simulink model "CBF_for_KinematicControl_UR3"  (R2024a)
settings: Solver=FixedStepAuto  StartTime=0.0  StopTime=Tf  FixedStep=Ts  RelTol=1e-3
undefined symbols (not defined in the file): config, d, InitAng, InitPos, lambda, Ts, x_obs
libraries: robotmaniplib x3, matrix_library x2, slctrl_constraint x1
settings Model: Creator=bumyong  LastModifiedBy=bumyong

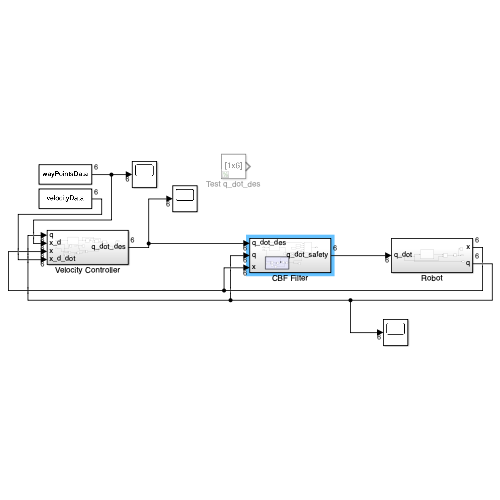
[thumbnail: Simulink's stored preview of the top-level diagram]
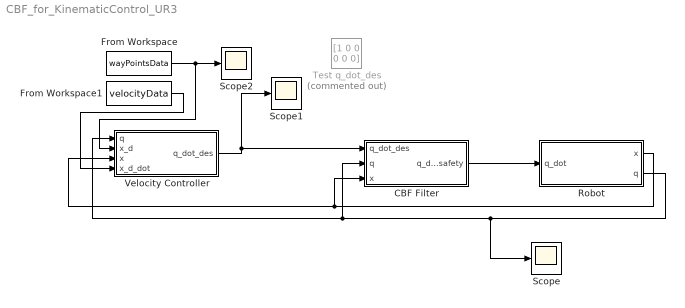
== system CBF_for_KinematicControl_UR3 ==
  CBF Filter : Subsystem
  From Workspace : FromWorkspace  VariableName=wayPointsData  Interpolate=off  OutputAfterFinalValue=Holding final value
  From Workspace1 : FromWorkspace  VariableName=velocityData  Interpolate=off  OutputAfterFinalValue=Holding final value
  Robot : Subsystem
  Scope : Scope
  Scope1 : Scope
  Scope2 : Scope
  Test q_dot_des : Constant  Commented=on  Value=[1 0 0 0 0 0]
  Velocity Controller : Subsystem
  wires:
  Robot/2(q) -> Scope/1, Velocity Controller/1(q), CBF Filter/2(q)
  Velocity Controller/1(q_dot_des) -> CBF Filter/1(q_dot_des), Scope1/1
  Robot/1(x) -> CBF Filter/3(x), Velocity Controller/3(x)
  From Workspace/1 -> Velocity Controller/2(x_d), Scope2/1
  From Workspace1/1 -> Velocity Controller/4(x_d_dot)
  CBF Filter/1(q_dot_safety) -> Robot/1(q_dot)

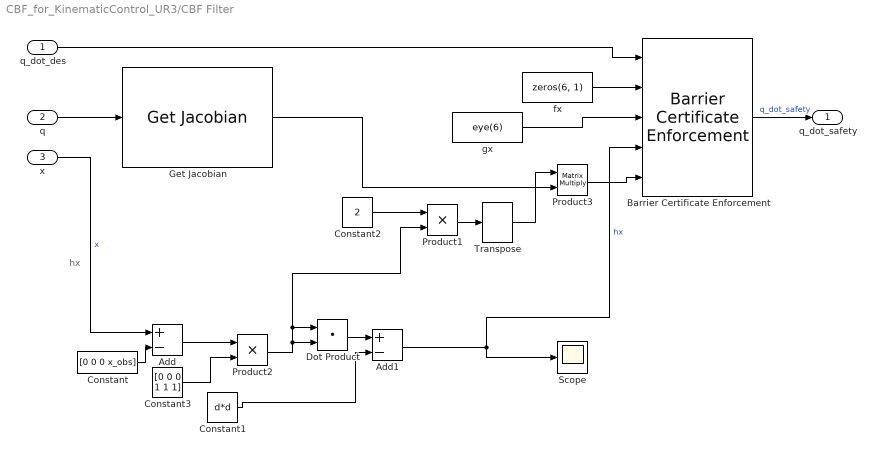
== system CBF_for_KinematicControl_UR3/CBF Filter ==
  note: hx
  q_dot_des : Inport
  q : Inport  Port=2
  x : Inport  Port=3
  Add : Sum  Inputs=+-
  Add1 : Sum  Inputs=+-
  Barrier Certificate Enforcement : slctrl_constraint/Barrier Certificate Enforcement  nx=6  nu=6  nc=1  gamma=gamma  beta=1  external_umax=off  external_umin=off  Ts=Ts  maxiter=200  tol=1e-6  output_exitflag=off
      settings: LibrarySourceBlock=slctrlblks/Constraint Control/Barrier Certificate Enforcement
  Constant : Constant  Value=[0 0 0 x_obs]
  Constant1 : Constant  Value=d*d
  Constant2 : Constant  Value=2
  Constant3 : Constant  Value=[0 0 0 1 1 1]
  Dot Product : DotProduct  OutDataTypeStr=Inherit: Inherit via internal rule
  Get Jacobian : robotmaniplib/Get Jacobian  RigidBodyTree=robot  EndEffector=tool0  SimulateUsing=Interpreted execution
  Product1 : Product
  Product2 : Product
  Product3 : Product  Multiplication=Matrix(*)
  Scope : Scope
  Transpose : matrix_library/Transpose
  fx : Constant  Value=zeros(6, 1)
  gx : Constant  Value=eye(6)
  q_dot_safety : Outport
  wires:
  q_dot_des/1 -> Barrier Certificate Enforcement/1
  fx/1 -> Barrier Certificate Enforcement/2
  Barrier Certificate Enforcement/1 -> q_dot_safety/1  "q_dot_safety"
  Add1/1 -> Barrier Certificate Enforcement/4, Scope/1  "hx"
  Dot Product/1 -> Add1/1
  Constant1/1 -> Add1/2
  Constant/1 -> Add/2
  q/1 -> Get Jacobian/1
  Constant2/1 -> Product1/1
  Product1/1 -> Transpose/1
  x/1 -> Add/1  "x"
  Add/1 -> Product2/1
  Product2/1 -> Dot Product/2, Product1/2, Dot Product/1
  Constant3/1 -> Product2/2
  gx/1 -> Barrier Certificate Enforcement/3
  Product3/1 -> Barrier Certificate Enforcement/5
  Transpose/1 -> Product3/1
  Get Jacobian/1 -> Product3/2

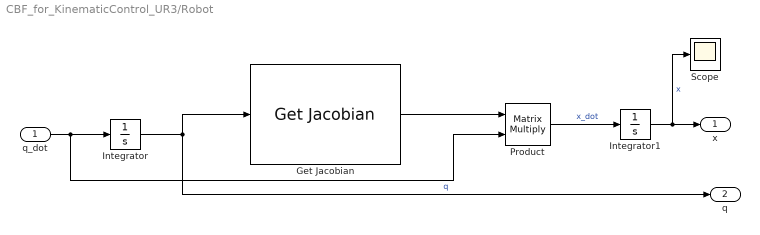
== system CBF_for_KinematicControl_UR3/Robot ==
  q_dot : Inport
  Get Jacobian : robotmaniplib/Get Jacobian  RigidBodyTree=robot  EndEffector=tool0  SimulateUsing=Interpreted execution
  Integrator : Integrator  InitialCondition=config
  Integrator1 : Integrator  InitialCondition=[InitAng, InitPos]
  Product : Product  Multiplication=Matrix(*)
  Scope : Scope
  x : Outport
  q : Outport  Port=2
  wires:
  q_dot/1 -> Product/2, Integrator/1
  Integrator/1 -> q/1, Get Jacobian/1  "q"
  Get Jacobian/1 -> Product/1
  Product/1 -> Integrator1/1  "x_dot"
  Integrator1/1 -> Scope/1, x/1  "x"

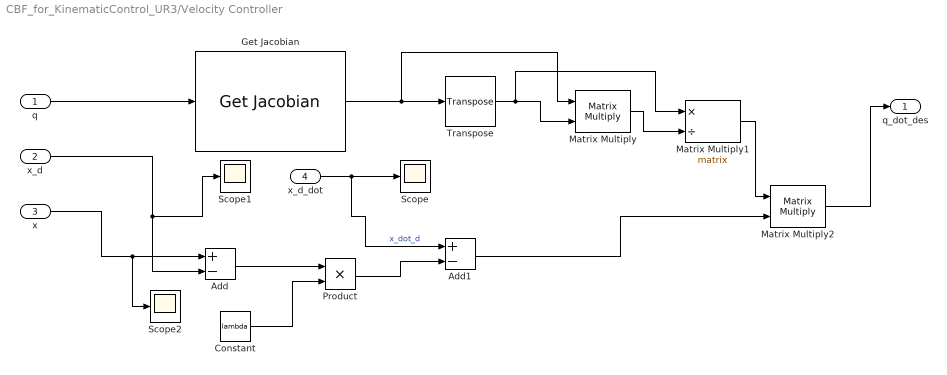
== system CBF_for_KinematicControl_UR3/Velocity Controller ==
  q : Inport
  x_d : Inport  Port=2
  x : Inport  Port=3
  x_d_dot : Inport  Port=4
  Add : Sum  Inputs=+-
  Add1 : Sum  Inputs=+-
  Constant : Constant  Value=lambda
  Get Jacobian : robotmaniplib/Get Jacobian  RigidBodyTree=robot  EndEffector=tool0  SimulateUsing=Interpreted execution
  Matrix Multiply : Product  Multiplication=Matrix(*)
  Matrix Multiply1 : Product  Inputs=*/  Multiplication=Matrix(*)
  Matrix Multiply2 : Product  Multiplication=Matrix(*)
  Product : Product
  Scope : Scope
  Scope1 : Scope
  Scope2 : Scope
  Transpose : matrix_library/Transpose
  q_dot_des : Outport
  wires:
  q/1 -> Get Jacobian/1
  Get Jacobian/1 -> Matrix Multiply/1, Transpose/1
  Transpose/1 -> Matrix Multiply1/1, Matrix Multiply/2
  Matrix Multiply/1 -> Matrix Multiply1/2
  x_d/1 -> Scope1/1, Add/2
  x/1 -> Scope2/1, Add/1
  Add/1 -> Product/1
  Constant/1 -> Product/2
  x_d_dot/1 -> Add1/1, Scope/1  "x_dot_d"
  Product/1 -> Add1/2
  Add1/1 -> Matrix Multiply2/2
  Matrix Multiply1/1 -> Matrix Multiply2/1
  Matrix Multiply2/1 -> q_dot_des/1
